simulink model "a2__AM_SSB"  (R2019a)
settings: Solver=VariableStepAuto  StartTime=0.0  StopTime=10.0  RelTol=1e-3
libraries: dsparch4 x2
settings Model: Creator=Thanh_Hai  LastModifiedBy=Thanh_Hai

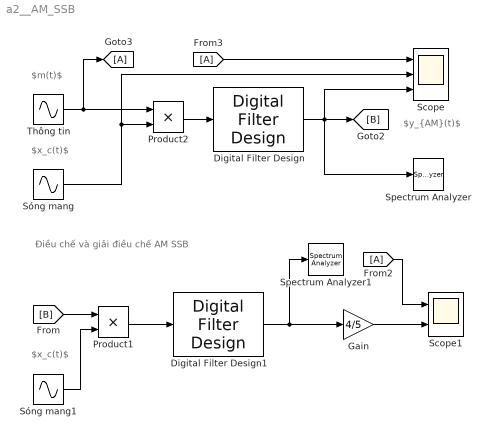
== system a2__AM_SSB ==
  note: $m(t)$
  note: $y_{AM}(t)$
  note: Điều chế và giải điều chế AM SSB
  note: $x_c(t)$
  note: $x_c(t)$
  Digital Filter Design : dsparch4/Digital Filter Design  mwdsp_browser_bugfix_var=off
  Digital Filter Design1 : dsparch4/Digital Filter Design  mwdsp_browser_bugfix_var=off
  Gain : Gain  Gain=4/5
  Product1 : Product
  Product2 : Product
  Scope : Scope  NumInputPorts=3
  Scope1 : Scope  NumInputPorts=2
  Spectrum Analyzer : SpectrumAnalyzer
  Spectrum Analyzer1 : SpectrumAnalyzer
  Sóng mang : Sin  Amplitude=5  Frequency=2*pi*5000  SampleTime=1/50000
  Sóng mang1 : Sin  Frequency=2*pi*5000  SampleTime=1/50000
  Thông tin : Sin  Frequency=2*pi*1000  SampleTime=1/50000
  wires:
  [A] -> Scope/1
  [A] -> Scope1/1
  Gain/1 -> Scope1/2
  [B] -> Product1/1
  Sóng mang/1 -> Scope/2, Product2/2
  Thông tin/1 -> Product2/1, [A]
  Sóng mang1/1 -> Product1/2
  Product2/1 -> Digital Filter Design/1
  Digital Filter Design/1 -> Scope/3, Spectrum Analyzer/1, [B]
  Product1/1 -> Digital Filter Design1/1
  Digital Filter Design1/1 -> Spectrum Analyzer1/1, Gain/1
